simulink model "controller_test_lqe"  (R2015a)
settings: Solver=FixedStepDiscrete  StartTime=0.0  StopTime=10  FixedStep=0.02  RelTol=1e-3
values from neighbouring files (symbols this model uses):
  B = 0.11    [signal_generation_acquisition.m]
  GAMMAE = B-Lc*C*B    [controller_design.m]
  PHIE = A-Lc*C*A    [controller_design.m]
undefined symbols (not defined in the file or in its folder): A, C, Lc
settings Model: ExtModeTrigDuration=200000  Creator=alunos  LastModifiedBy=jmgri
settings DataIOCC: LimitDataPoints=off
settings HardwareCC: ProdBitPerPointer=64  ProdLargestAtomicFloat=Float  ProdIntDivRoundTo=Zero  ProdEndianess=LittleEndian  ProdHWDeviceType=Specified  TargetIntDivRoundTo=Zero  TargetEndianess=LittleEndian  TargetHWDeviceType=Intel->x86/Pentium
settings RTWCC: SystemTargetFile=rtwin.tlc  TemplateMakefile=rtwin.tmf  Description=Simulink Desktop Real-Time  RTWCompilerOptimization=on
settings CodeAppCC: MaxIdLength=95
settings RTWinTargetCC: TargetPreCompLibLocation=C:\Program Files\MATLAB\R2017a\toolbox\sldrt\lib\win64  GeneratePreprocessorConditionals=Use local settings  ExtModeMexFile=sldrtext

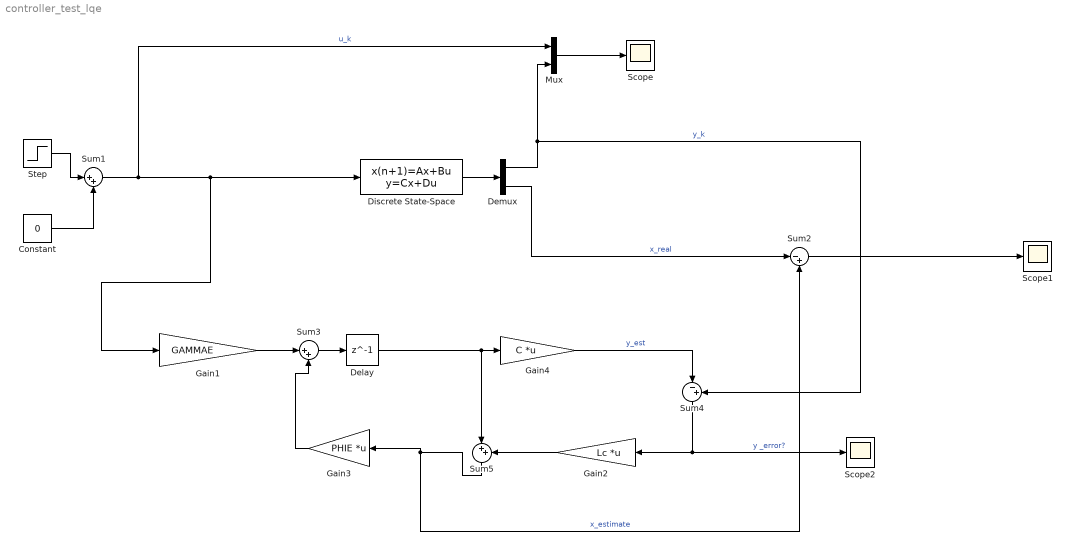
== system controller_test_lqe ==
  Constant : Constant  Value=0
  Delay : Delay  DelayLength=1
  Demux : Demux  Outputs=[1 length(A)]
  Discrete State-Space : DiscreteStateSpace  A=A  B=B  C=[C;eye(length(A))]  D=[0;zeros(length(A),1)]  SampleTime=-1
  Gain1 : Gain  Gain=GAMMAE
  Gain2 : Gain  Gain=Lc  Multiplication=Matrix(K*u)
  Gain3 : Gain  Gain=PHIE  Multiplication=Matrix(K*u)
  Gain4 : Gain  Gain=C  Multiplication=Matrix(K*u)
  Mux : Mux  Inputs=2
  Scope : Scope
      settings: TickLabels=on  SaveName=simulation_data  SampleInput=on
  Scope1 : Scope
      settings: TickLabels=on  SaveName=simulation_data1  SampleInput=on
  Scope2 : Scope
      settings: TickLabels=on  SaveName=simulation_data2  SampleInput=on
  Step : Step  Before=1  After=0  SampleTime=0.02
  Sum1 : Sum  Inputs=|++
  Sum2 : Sum  Inputs=|-+
  Sum3 : Sum  Inputs=|++
  Sum4 : Sum  Inputs=|-+
  Sum5 : Sum  Inputs=|++
  wires:
  Mux/1 -> Scope/1
  Discrete State-Space/1 -> Demux/1
  Step/1 -> Sum1/1
  Constant/1 -> Sum1/2
  Demux/2 -> Sum2/1  "x_real"
  Sum2/1 -> Scope1/1
  Sum1/1 -> Mux/1, Gain1/1, Discrete State-Space/1  "u_k"
  Gain1/1 -> Sum3/1
  Sum3/1 -> Delay/1
  Delay/1 -> Gain4/1, Sum5/1
  Sum4/1 -> Scope2/1, Gain2/1  "y _error?"
  Gain2/1 -> Sum5/2
  Gain3/1 -> Sum3/2
  Demux/1 -> Sum4/2, Mux/2  "y_k"
  Sum5/1 -> Gain3/1, Sum2/2  "x_estimate"
  Gain4/1 -> Sum4/1  "y_est"
